simulink model "Test_with_WMM"  (Simulink 7.3)
settings: Solver=ode45  StartTime=0.0  StopTime=7200  RelTol=1e-3
libraries: simulink x2, aerolib6dof2 x1, vrlib x1, aerolibgravity2 x1
settings Model: Creator=Deepti  LastModifiedBy=Owner
settings OptimizationCC: InitFltsAndDblsToZero=on
settings DebuggingCC: SaveWithParameterizedLinksMsg=none
settings GRTTargetCC: TargetFcnLib=ansi_tfl_tmw.mat

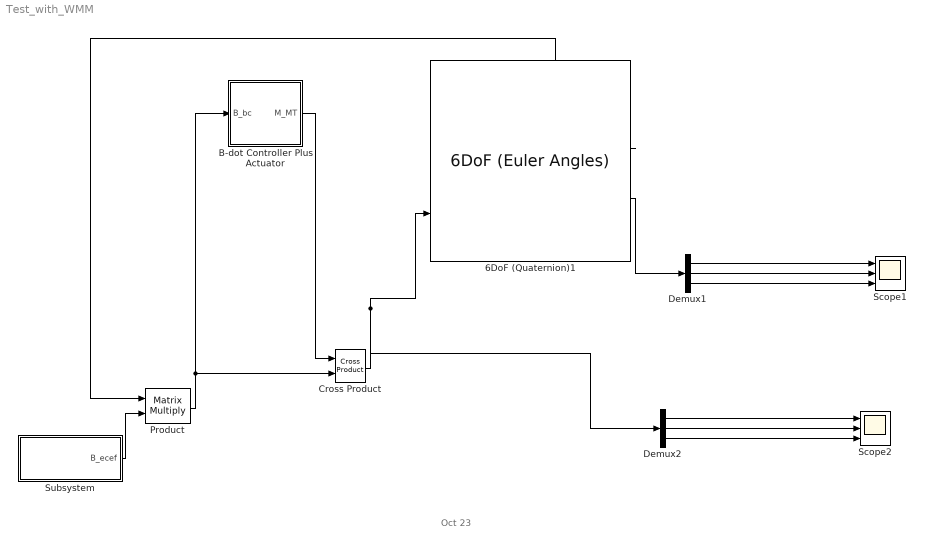
== system Test_with_WMM ==
  note: Oct 23
  6DoF (Quaternion)1 : aerolib6dof2/6DoF (Euler Angles)  SystemSampleTime=-1  units=Metric (MKS)  mtype=Fixed  rep=Euler Angles  xme_0=[0 0 0]  Vm_0=[0 0 0]  eul_0=[0 0 0]  pm_0=[.2 .3 .1]  mass_0=10.0  mass_e=0  mass_f=0  inertia=[1 0 0; 0 1 0; 0 0 2]  inertia_e=eye(3)  inertia_f=eye(3)  k_quat=1.0
  B-dot Controller Plus Actuator : Subsystem
  Cross Product : vrlib/Utilities/Cross Product  SystemSampleTime=-1
  Demux1 : Demux  Outputs=3
  Demux2 : Demux  Outputs=3
  Product : Product  Multiplication=Matrix(*)  OutDataType=fixdt(1, 16)  OutScaling=2^0  RndMeth=Zero
  Scope1 : Scope  NumInputPorts=3
      settings: YMin=-450000~-450000~226550  YMax=450000~450000~227300
  Scope2 : Scope  NumInputPorts=3
      settings: YMin=-450000~-450000~226550  YMax=450000~450000~227300  SaveName=ScopeData9
  Subsystem : Subsystem
  wires:
  6DoF (Quaternion)1/6 -> Demux1/1
  Subsystem/1(B_ecef) -> Product/2
  6DoF (Quaternion)1/4 -> Product/1
  Product/1 -> B-dot Controller Plus Actuator/1(B_bc), Cross Product/2
  B-dot Controller Plus Actuator/1(M_MT) -> Cross Product/1
  Cross Product/1 -> 6DoF (Quaternion)1/2, Demux2/1
  Demux1/1 -> Scope1/1
  Demux1/2 -> Scope1/2
  Demux1/3 -> Scope1/3
  Demux2/1 -> Scope2/1
  Demux2/2 -> Scope2/2
  Demux2/3 -> Scope2/3

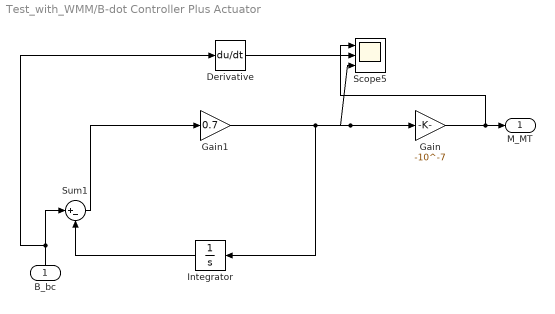
== system Test_with_WMM/B-dot Controller Plus Actuator ==
  B_bc : Inport  OutDataType=sfix(16)  OutScaling=2^0
  Derivative : Derivative
  Gain : Gain  Gain=-10^-7  ParameterDataType=fixdt(1, 16)  ParameterScaling=2^0  OutDataType=fixdt(1, 16)  OutScaling=2^0
  Gain1 : Gain  Gain=0.7  ParameterDataType=fixdt(1, 16)  ParameterScaling=2^0  OutDataType=fixdt(1, 16)  OutScaling=2^0
  Integrator : Integrator
  Scope5 : Scope  NumInputPorts=3
      settings: YMin=-1.5e+006~-5~-5  YMax=1.5e+006~5~5  SaveName=ScopeData5
  Sum1 : Sum  Inputs=|+-  OutDataType=fixdt(1, 16)  OutScaling=2^0
  M_MT : Outport  OutDataType=sfix(16)  OutScaling=2^0
  wires:
  Sum1/1 -> Gain1/1
  Gain1/1 -> Integrator/1, Gain/1, Scope5/3
  Integrator/1 -> Sum1/2
  Gain/1 -> Scope5/2, M_MT/1
  Derivative/1 -> Scope5/1
  B_bc/1 -> Sum1/1, Derivative/1

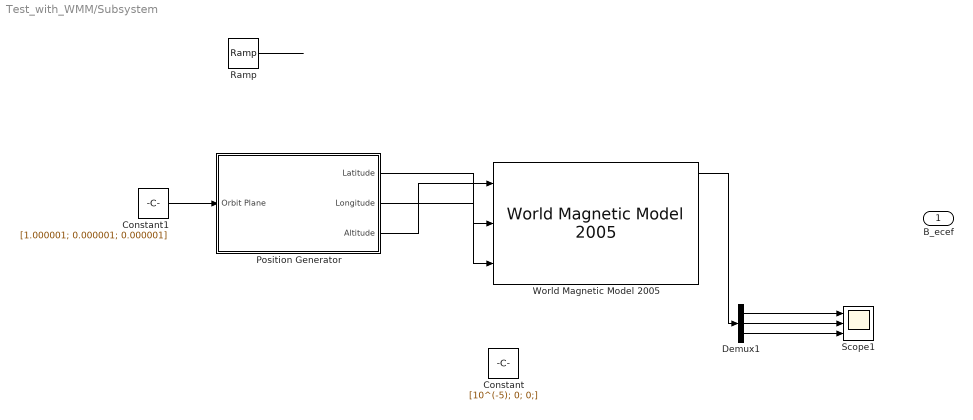
== system Test_with_WMM/Subsystem ==
  Constant : Constant  Value=[10^(-5); 0; 0;]  OutDataType=sfix(16)  OutScaling=2^0
  Constant1 : Constant  Value=[1.000001; 0.000001; 0.000001]  VectorParams1D=off  OutDataType=sfix(16)  OutScaling=2^0
  Demux1 : Demux  Outputs=3
  Position Generator : Subsystem  mask{omega_0=2*pi, h=700000, lat_init=0, long_init=0}
      mask prompts: omega_0 "Orbital frequency (orbits/second)"; h "Orbit height (m)"; lat_init "Initial Latitude (deg)"; long_init "Initial Longitude (deg)"
  Ramp : simulink/Sources/Ramp  SystemSampleTime=-1  slope=1  start=0  X0=0
  Scope1 : Scope  NumInputPorts=3
      settings: YMin=2000~-9000~-45000  YMax=21000~6000~15000  SaveName=Magnetic_Field  MaxDataPoints=72000  SampleInput=on  SampleTime=0.1
  World Magnetic Model 2005 : aerolibgravity2/World Magnetic Model 2005  SystemSampleTime=-1  units=Metric (MKS)  time_in=off  month=January  day=1  year=2005  action=Error  h_out=on  dec_out=on  inc_out=on  ti_out=on
  B_ecef : Outport  OutDataType=sfix(16)  OutScaling=2^0
  wires:
  World Magnetic Model 2005/1 -> Demux1/1
  Position Generator/3(Altitude) -> World Magnetic Model 2005/1
  Position Generator/1(Latitude) -> World Magnetic Model 2005/2
  Position Generator/2(Longitude) -> World Magnetic Model 2005/3
  Constant1/1 -> Position Generator/1(Orbit Plane)
  Ramp/1 -> ?
  Demux1/1 -> Scope1/1
  Demux1/2 -> Scope1/2
  Demux1/3 -> Scope1/3

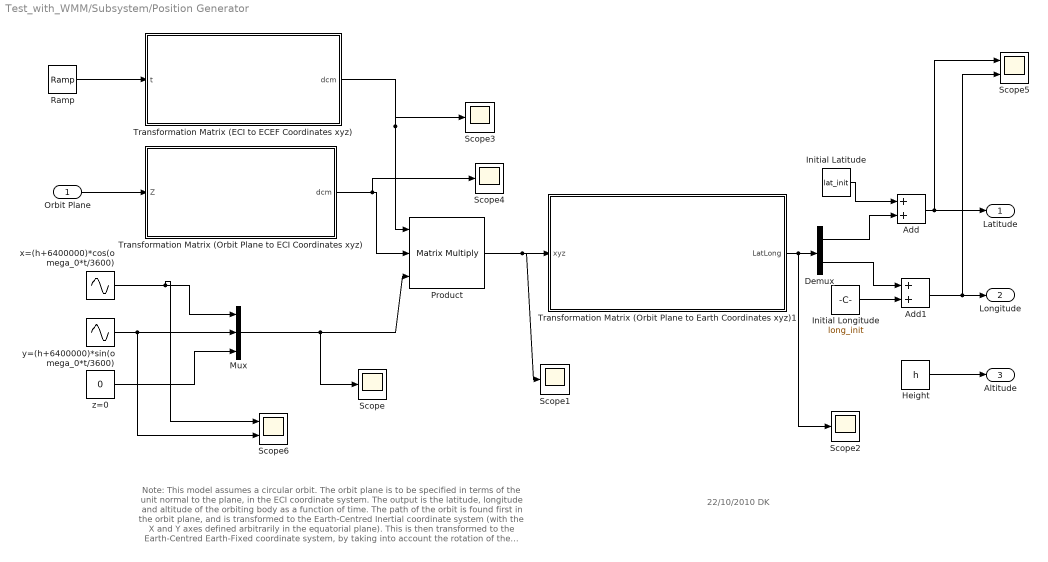
== system Test_with_WMM/Subsystem/Position Generator ==
  note: Note: This model assumes a circular orbit. The orbit plane is to be specified in terms of the unit normal to the plane, in the ECI coordinate system.
      | The output is the latitude, longitude and altitude of the orbiting body as a function of time. The path of the orbit is found first in the orbit plane, and
      |        is transformed to the Earth-Centred Inertial coordinate system (with the X and Y axes defined arbitrarily in the equatorial plane). This is then transformed
      | to the Earth-Centred Earth-Fixed coordinate system, by taking into account the rotation of the Earth.
  note: 22/10/2010
      | DK
  Orbit Plane : Inport  OutDataType=sfix(16)  OutScaling=2^0
  Add : Sum  OutDataType=sfix(16)  OutScaling=2^-10
  Add1 : Sum  OutDataType=sfix(16)  OutScaling=2^-10
  Demux : Demux  Outputs=2
  Height : Constant  Value=h  OutDataType=sfix(16)  OutScaling=2^0
  Initial Latitude : Constant  Value=lat_init  OutDataType=sfix(16)  OutScaling=2^0
  Initial Longitude : Constant  Value=long_init  OutDataType=sfix(16)  OutScaling=2^0
  Mux : Mux  Inputs=3
  Product : Product  Inputs=3  Multiplication=Matrix(*)  OutDataType=sfix(16)  OutScaling=2^0  RndMeth=Zero
  Ramp : simulink/Sources/Ramp  SystemSampleTime=-1  slope=1  start=0  X0=0
  Scope{,1..4} (5 alike) : Scope
      Scope1 settings: SaveName=ScopeData2
      Scope2 settings: SaveName=ScopeData3
      Scope3 settings: SaveName=ScopeData5
      Scope4 settings: SaveName=ScopeData6
  Scope5 : Scope  NumInputPorts=2
      settings: YMin=-5~-5  YMax=5~5  SaveName=ScopeData7
  Scope6 : Scope  NumInputPorts=2
      settings: YMin=-5~-5  YMax=5~5  SaveName=ScopeData8
  Transformation Matrix (ECI to ECEF Coordinates xyz) : Stateflow chart
  Transformation Matrix (Orbit Plane to ECI Coordinates xyz) : Stateflow chart
  Transformation Matrix (Orbit Plane to Earth Coordinates xyz)1 : Stateflow chart
  x=(h+6400000)*cos(omega_0*t/3600) : Sin  Amplitude=h+6400000  Bias=0  Frequency=omega_0/7200  Phase=pi/2  Samples=10  SampleTime=0  Offset=0
  y=(h+6400000)*sin(omega_0*t/3600) : Sin  Amplitude=h+6400000  Bias=0  Frequency=omega_0/7200  Phase=0  Samples=10  SampleTime=0  Offset=0
  z=0 : Constant  Value=0  OutDataType=sfix(16)  OutScaling=2^0
  Latitude : Outport  OutDataType=sfix(16)  OutScaling=2^0
  Longitude : Outport  Port=2  OutDataType=sfix(16)  OutScaling=2^0
  Altitude : Outport  Port=3  OutDataType=sfix(16)  OutScaling=2^0
  wires:
  Orbit Plane/1 -> Transformation Matrix (Orbit Plane to ECI Coordinates xyz)/1(Z)
  x=(h+6400000)*cos(omega_0*t/3600)/1 -> Mux/1, Scope6/1
  y=(h+6400000)*sin(omega_0*t/3600)/1 -> Mux/2, Scope6/2
  z=0/1 -> Mux/3
  Mux/1 -> Scope/1, Product/3
  Transformation Matrix (Orbit Plane to ECI Coordinates xyz)/1(dcm) -> Product/2, Scope4/1
  Height/1 -> Altitude/1
  Product/1 -> Transformation Matrix (Orbit Plane to Earth Coordinates xyz)1/1(xyz), Scope1/1
  Transformation Matrix (Orbit Plane to Earth Coordinates xyz)1/1(LatLong) -> Demux/1, Scope2/1
  Demux/1 -> Add/2
  Demux/2 -> Add1/1
  Initial Latitude/1 -> Add/1
  Add/1 -> Latitude/1, Scope5/1
  Initial Longitude/1 -> Add1/2
  Add1/1 -> Longitude/1, Scope5/2
  Ramp/1 -> Transformation Matrix (ECI to ECEF Coordinates xyz)/1(t)
  Transformation Matrix (ECI to ECEF Coordinates xyz)/1(dcm) -> Product/1, Scope3/1

== matlab function Subsystem/Position Generator/Transformation Matrix (Orbit Plane to ECI Coordinates xyz) ==
  data: dcm output double; Z input double
function dcm = orbit_plane_to_ECI(Z)
% This block supports an embeddable subset of the MATLAB language.
% See the help menu for details. 
%X=[1;0;0]-(Z'*[1;0;0])*Z;
X=[0; 0; 0];
X(1,1)=1;
X(2,1)=1;
X(3,1)=(-Z(1)*X(1)-Z(2)*X(2))/Z(3);
X=X./norm(X);
Y=cross(Z,X);
dcm=[X Y Z];
end

== matlab function Subsystem/Position Generator/Transformation Matrix (Orbit Plane to Earth Coordinates xyz)1 ==
  data: LatLong output double; xyz input double
function LatLong = Find_Latitude_and_Longitude(xyz)
% This block supports an embeddable subset of the MATLAB language.
% See the help menu for details. 
longitude=atand(xyz(2,1)/xyz(1,1));  %atand(y/x)
latitude=asind(xyz(3,1)/norm(xyz));
LatLong=[latitude; longitude];
end

== matlab function Subsystem/Position Generator/Transformation Matrix (ECI to ECEF Coordinates xyz) ==
  data: dcm output double; t input double
function dcm = ECI_to_ECEF(t)
% This block supports an embeddable subset of the MATLAB language.
% See the help menu for details. 
omega_earth=0/(3600*24);
dcm=[cos(omega_earth*t) sin(omega_earth*t) 0;-sin(omega_earth*t) cos(omega_earth*t) 0; 0 0 1];
end
